simulink model "matlab_ros_com"  (R2017b)
settings: Solver=VariableStepAuto  StartTime=0.0  StopTime=inf  FixedStep=0.001  RelTol=1e-3  EnableMultiTasking=on
InitFcn:
  | sub_pose_time=0.1;
  | sub_vel_time=0.1;
  | pub_vel_time=0.1;
  | pub_pose_time=0.1;
undefined symbols (not defined in the file or in its folder): Pose, Twist
libraries: robotlib x28, simulink x5
settings Model: Creator=Administrator  LastModifiedBy=shitou
settings OptimizationCC: LifeSpan=inf
settings DebuggingCC: SFUnexpectedBacktrackingDiag=warning  SFNoUnconditionalDefaultTransitionDiag=warning  SFExecutionAtInitializationDiag=none
settings CodeAppCC: StateflowObjectComments=on
settings GRTTargetCC: TargetLangStandard=C89/C90 (ANSI)  GeneratePreprocessorConditionals=Disable all
settings ConfigComp: CovMetricSettings=dw  CovHtmlReporting=on  CovSaveCumulativeToWorkspaceVar=on  CovSaveSingleToWorkspaceVar=on  CovExternalEMLEnable=off

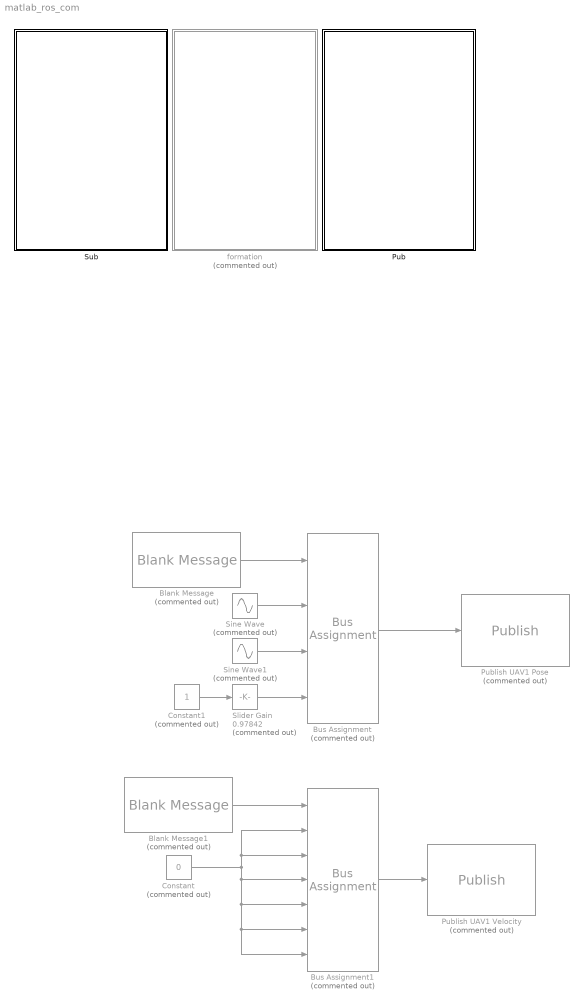
== system matlab_ros_com ==
  Blank Message : robotlib/Blank Message  Commented=on  SourceLibraryInfo=This block requires Robotics System Toolbox  messageType=geometry_msgs/PoseStamped  SampleTime=-1
      settings: SourceProductBaseCode=RO
  Blank Message1 : robotlib/Blank Message  Commented=on  SourceLibraryInfo=This block requires Robotics System Toolbox  messageType=geometry_msgs/TwistStamped  SampleTime=inf
      settings: SourceProductBaseCode=RO
  Bus Assignment : BusAssignment  Commented=on  AssignedSignals=Pose.Position.X,Pose.Position.Y,Pose.Position.Z
  Bus Assignment1 : BusAssignment  Commented=on  AssignedSignals=Twist.Linear.X,Twist.Linear.Y,Twist.Linear.Z,Twist.Angular.X,Twist.Angular.Y,Twist.Angular.Z
  Constant : Constant  Commented=on  Value=0
  Constant1 : Constant  Commented=on
  Pub : Subsystem
  Publish UAV1 Pose : robotlib/Publish  Commented=on  SourceLibraryInfo=This block requires Robotics System Toolbox  topicSource=Specify your own  topic=uav1_matlab/mavros/local_position/pose  messageType=geometry_msgs/PoseStamped  messageQueueLength=1
      settings: SourceProductBaseCode=RO
  Publish UAV1 Velocity : robotlib/Publish  Commented=on  SourceLibraryInfo=This block requires Robotics System Toolbox  topicSource=Specify your own  topic=uav1_matlab/mavros/local_position/velocity_local  messageType=geometry_msgs/TwistStamped  messageQueueLength=1
      settings: SourceProductBaseCode=RO
  Sine Wave : Sin  Commented=on  Frequency=0.05*pi
  Sine Wave1 : Sin  Commented=on  Frequency=0.05*pi  Phase=pi/2
  Slider Gain : simulink/Math Operations/Slider Gain  Commented=on  gain=0.97842  low=0  high=2
  Sub : Subsystem
  formation : Subsystem  Commented=on
  wires:
  Blank Message/1 -> Bus Assignment/1
  Bus Assignment/1 -> Publish UAV1 Pose/1
  Blank Message1/1 -> Bus Assignment1/1
  Bus Assignment1/1 -> Publish UAV1 Velocity/1
  Constant1/1 -> Slider Gain/1
  Slider Gain/1 -> Bus Assignment/4
  Sine Wave/1 -> Bus Assignment/2
  Sine Wave1/1 -> Bus Assignment/3
  Constant/1 -> Bus Assignment1/7, Bus Assignment1/6, Bus Assignment1/5, Bus Assignment1/4, Bus Assignment1/3, Bus Assignment1/2

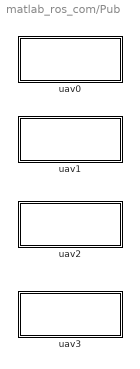
== system matlab_ros_com/Pub ==
  uav0 : Subsystem
  uav1 : Subsystem
  uav2 : Subsystem
  uav3 : Subsystem

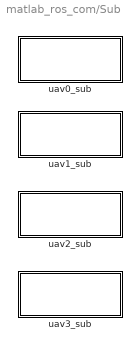
== system matlab_ros_com/Sub ==
  uav0_sub : Subsystem
  uav1_sub : Subsystem
  uav2_sub : Subsystem
  uav3_sub : Subsystem

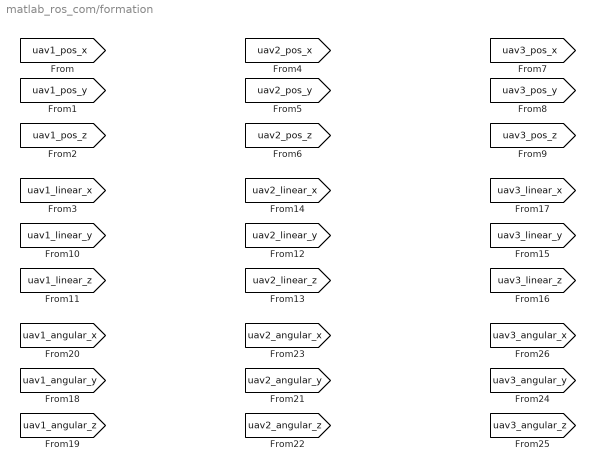
== system matlab_ros_com/formation ==

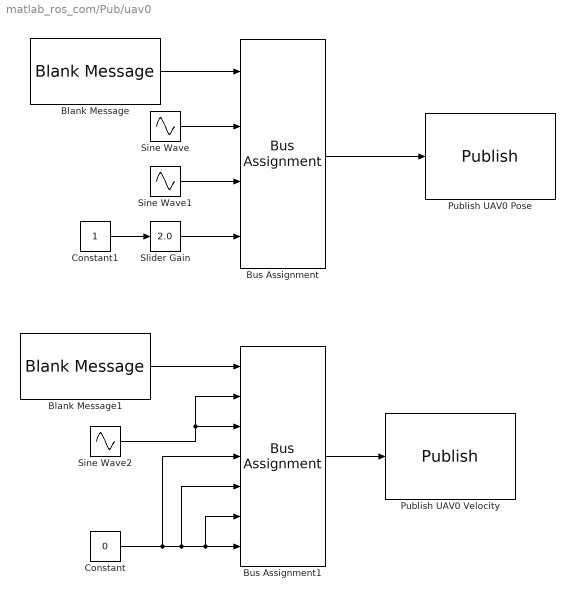
== system matlab_ros_com/Pub/uav0 ==
  Blank Message : robotlib/Blank Message  SourceLibraryInfo=This block requires Robotics System Toolbox  messageType=geometry_msgs/PoseStamped  SampleTime=pub_pose_time
      settings: SourceProductBaseCode=RO
  Blank Message1 : robotlib/Blank Message  SourceLibraryInfo=This block requires Robotics System Toolbox  messageType=geometry_msgs/TwistStamped  SampleTime=-1
      settings: SourceProductBaseCode=RO
  Bus Assignment : BusAssignment  AssignedSignals=Pose.Position.X,Pose.Position.Y,Pose.Position.Z
  Bus Assignment1 : BusAssignment  AssignedSignals=Twist.Linear.X,Twist.Linear.Y,Twist.Linear.Z,Twist.Angular.X,Twist.Angular.Y,Twist.Angular.Z
  Constant : Constant  Value=0  SampleTime=pub_vel_time
  Constant1 : Constant  SampleTime=pub_pose_time
  Publish UAV0 Pose : robotlib/Publish  SourceLibraryInfo=This block requires Robotics System Toolbox  topicSource=Specify your own  topic=uav0_matlab/mavros/local_position/pose  messageType=geometry_msgs/PoseStamped  messageQueueLength=1
      settings: SourceProductBaseCode=RO
  Publish UAV0 Velocity : robotlib/Publish  SourceLibraryInfo=This block requires Robotics System Toolbox  topicSource=Specify your own  topic=uav0_matlab/mavros/local_position/velocity_local  messageType=geometry_msgs/TwistStamped  messageQueueLength=1
      settings: SourceProductBaseCode=RO
  Sine Wave : Sin  Amplitude=10  Frequency=0.1*pi
  Sine Wave1 : Sin  Amplitude=10  Frequency=0.1*pi  Phase=pi/2
  Sine Wave2 : Sin  Frequency=0.1*pi  Phase=pi/2
  Slider Gain : simulink/Math Operations/Slider Gain  gain=2.0  low=0  high=2
  wires:
  Blank Message/1 -> Bus Assignment/1
  Bus Assignment/1 -> Publish UAV0 Pose/1
  Blank Message1/1 -> Bus Assignment1/1
  Bus Assignment1/1 -> Publish UAV0 Velocity/1
  Constant1/1 -> Slider Gain/1
  Slider Gain/1 -> Bus Assignment/4
  Sine Wave/1 -> Bus Assignment/2
  Sine Wave1/1 -> Bus Assignment/3
  Constant/1 -> Bus Assignment1/4, Bus Assignment1/5, Bus Assignment1/6, Bus Assignment1/7
  Sine Wave2/1 -> Bus Assignment1/3, Bus Assignment1/2

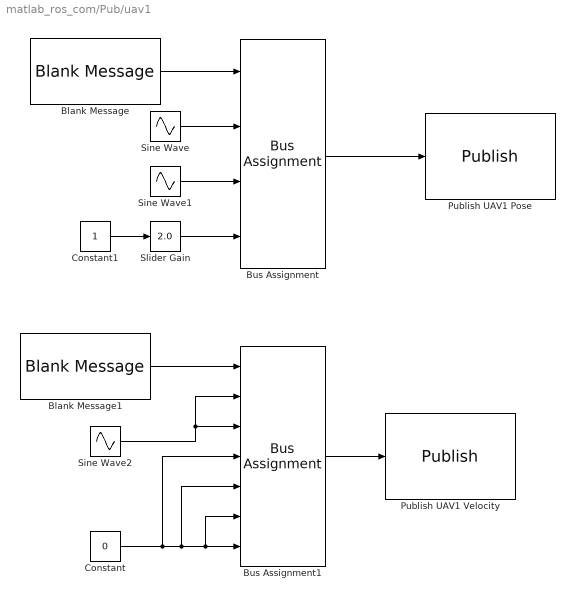
== system matlab_ros_com/Pub/uav1 ==
  Blank Message : robotlib/Blank Message  SourceLibraryInfo=This block requires Robotics System Toolbox  messageType=geometry_msgs/PoseStamped  SampleTime=pub_pose_time
      settings: SourceProductBaseCode=RO
  Blank Message1 : robotlib/Blank Message  SourceLibraryInfo=This block requires Robotics System Toolbox  messageType=geometry_msgs/TwistStamped  SampleTime=-1
      settings: SourceProductBaseCode=RO
  Bus Assignment : BusAssignment  AssignedSignals=Pose.Position.X,Pose.Position.Y,Pose.Position.Z
  Bus Assignment1 : BusAssignment  AssignedSignals=Twist.Linear.X,Twist.Linear.Y,Twist.Linear.Z,Twist.Angular.X,Twist.Angular.Y,Twist.Angular.Z
  Constant : Constant  Value=0  SampleTime=pub_vel_time
  Constant1 : Constant  SampleTime=pub_pose_time
  Publish UAV1 Pose : robotlib/Publish  SourceLibraryInfo=This block requires Robotics System Toolbox  topicSource=Specify your own  topic=uav1_matlab/mavros/local_position/pose  messageType=geometry_msgs/PoseStamped  messageQueueLength=1
      settings: SourceProductBaseCode=RO
  Publish UAV1 Velocity : robotlib/Publish  SourceLibraryInfo=This block requires Robotics System Toolbox  topicSource=Specify your own  topic=uav1_matlab/mavros/local_position/velocity_local  messageType=geometry_msgs/TwistStamped  messageQueueLength=1
      settings: SourceProductBaseCode=RO
  Sine Wave : Sin  Amplitude=10  Frequency=0.1*pi
  Sine Wave1 : Sin  Amplitude=10  Frequency=0.1*pi  Phase=pi/2
  Sine Wave2 : Sin  Frequency=0.1*pi  Phase=pi/2
  Slider Gain : simulink/Math Operations/Slider Gain  gain=2.0  low=0  high=2
  wires:
  Blank Message/1 -> Bus Assignment/1
  Bus Assignment/1 -> Publish UAV1 Pose/1
  Blank Message1/1 -> Bus Assignment1/1
  Bus Assignment1/1 -> Publish UAV1 Velocity/1
  Constant1/1 -> Slider Gain/1
  Slider Gain/1 -> Bus Assignment/4
  Sine Wave/1 -> Bus Assignment/2
  Sine Wave1/1 -> Bus Assignment/3
  Constant/1 -> Bus Assignment1/4, Bus Assignment1/5, Bus Assignment1/6, Bus Assignment1/7
  Sine Wave2/1 -> Bus Assignment1/3, Bus Assignment1/2

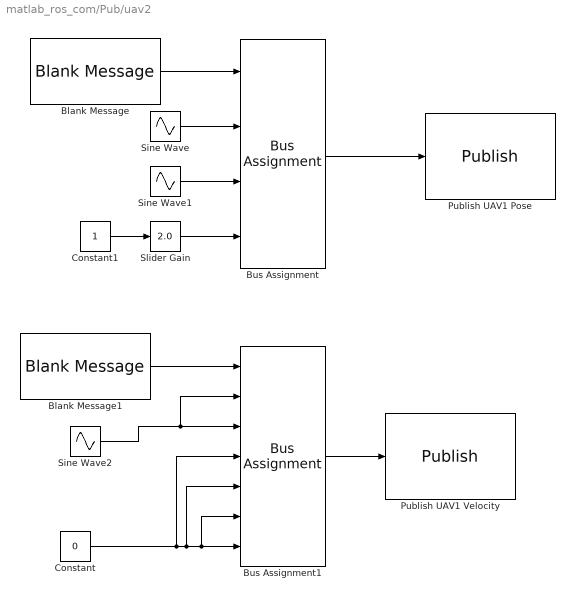
== system matlab_ros_com/Pub/uav2 ==
  Blank Message : robotlib/Blank Message  SourceLibraryInfo=This block requires Robotics System Toolbox  messageType=geometry_msgs/PoseStamped  SampleTime=pub_pose_time
      settings: SourceProductBaseCode=RO
  Blank Message1 : robotlib/Blank Message  SourceLibraryInfo=This block requires Robotics System Toolbox  messageType=geometry_msgs/TwistStamped  SampleTime=pub_vel_time
      settings: SourceProductBaseCode=RO
  Bus Assignment : BusAssignment  AssignedSignals=Pose.Position.X,Pose.Position.Y,Pose.Position.Z
  Bus Assignment1 : BusAssignment  AssignedSignals=Twist.Linear.X,Twist.Linear.Y,Twist.Linear.Z,Twist.Angular.X,Twist.Angular.Y,Twist.Angular.Z
  Constant : Constant  Value=0  SampleTime=pub_vel_time
  Constant1 : Constant  SampleTime=pub_pose_time
  Publish UAV1 Pose : robotlib/Publish  SourceLibraryInfo=This block requires Robotics System Toolbox  topicSource=Specify your own  topic=uav2_matlab/mavros/local_position/pose  messageType=geometry_msgs/PoseStamped  messageQueueLength=1
      settings: SourceProductBaseCode=RO
  Publish UAV1 Velocity : robotlib/Publish  SourceLibraryInfo=This block requires Robotics System Toolbox  topicSource=Specify your own  topic=uav2_matlab/mavros/local_position/velocity_local  messageType=geometry_msgs/TwistStamped  messageQueueLength=1
      settings: SourceProductBaseCode=RO
  Sine Wave : Sin  Amplitude=10  Frequency=0.1*pi
  Sine Wave1 : Sin  Amplitude=10  Frequency=0.1*pi  Phase=pi/2
  Sine Wave2 : Sin  Frequency=0.1*pi  Phase=pi/2
  Slider Gain : simulink/Math Operations/Slider Gain  gain=2.0  low=0  high=2
  wires:
  Blank Message/1 -> Bus Assignment/1
  Bus Assignment/1 -> Publish UAV1 Pose/1
  Blank Message1/1 -> Bus Assignment1/1
  Bus Assignment1/1 -> Publish UAV1 Velocity/1
  Constant1/1 -> Slider Gain/1
  Slider Gain/1 -> Bus Assignment/4
  Sine Wave/1 -> Bus Assignment/2
  Sine Wave1/1 -> Bus Assignment/3
  Constant/1 -> Bus Assignment1/4, Bus Assignment1/5, Bus Assignment1/6, Bus Assignment1/7
  Sine Wave2/1 -> Bus Assignment1/2, Bus Assignment1/3

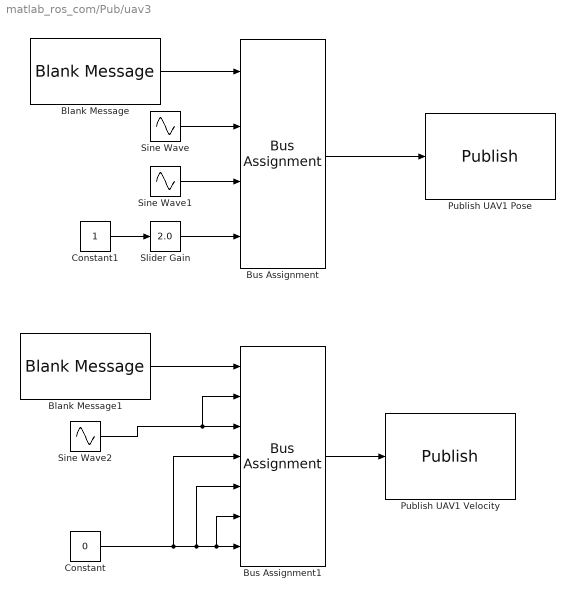
== system matlab_ros_com/Pub/uav3 ==
  Blank Message : robotlib/Blank Message  SourceLibraryInfo=This block requires Robotics System Toolbox  messageType=geometry_msgs/PoseStamped  SampleTime=pub_pose_time
      settings: SourceProductBaseCode=RO
  Blank Message1 : robotlib/Blank Message  SourceLibraryInfo=This block requires Robotics System Toolbox  messageType=geometry_msgs/TwistStamped  SampleTime=pub_vel_time
      settings: SourceProductBaseCode=RO
  Bus Assignment : BusAssignment  AssignedSignals=Pose.Position.X,Pose.Position.Y,Pose.Position.Z
  Bus Assignment1 : BusAssignment  AssignedSignals=Twist.Linear.X,Twist.Linear.Y,Twist.Linear.Z,Twist.Angular.X,Twist.Angular.Y,Twist.Angular.Z
  Constant : Constant  Value=0  SampleTime=pub_vel_time
  Constant1 : Constant  SampleTime=pub_pose_time
  Publish UAV1 Pose : robotlib/Publish  SourceLibraryInfo=This block requires Robotics System Toolbox  topicSource=Specify your own  topic=uav3_matlab/mavros/local_position/pose  messageType=geometry_msgs/PoseStamped  messageQueueLength=1
      settings: SourceProductBaseCode=RO
  Publish UAV1 Velocity : robotlib/Publish  SourceLibraryInfo=This block requires Robotics System Toolbox  topicSource=Specify your own  topic=uav3_matlab/mavros/local_position/velocity_local  messageType=geometry_msgs/TwistStamped  messageQueueLength=1
      settings: SourceProductBaseCode=RO
  Sine Wave : Sin  Amplitude=10  Frequency=0.1*pi
  Sine Wave1 : Sin  Amplitude=10  Frequency=0.1*pi  Phase=pi/2
  Sine Wave2 : Sin  Frequency=0.1*pi  Phase=pi/2
  Slider Gain : simulink/Math Operations/Slider Gain  gain=2.0  low=0  high=2
  wires:
  Blank Message/1 -> Bus Assignment/1
  Bus Assignment/1 -> Publish UAV1 Pose/1
  Blank Message1/1 -> Bus Assignment1/1
  Bus Assignment1/1 -> Publish UAV1 Velocity/1
  Constant1/1 -> Slider Gain/1
  Slider Gain/1 -> Bus Assignment/4
  Sine Wave/1 -> Bus Assignment/2
  Sine Wave1/1 -> Bus Assignment/3
  Constant/1 -> Bus Assignment1/4, Bus Assignment1/5, Bus Assignment1/6, Bus Assignment1/7
  Sine Wave2/1 -> Bus Assignment1/2, Bus Assignment1/3

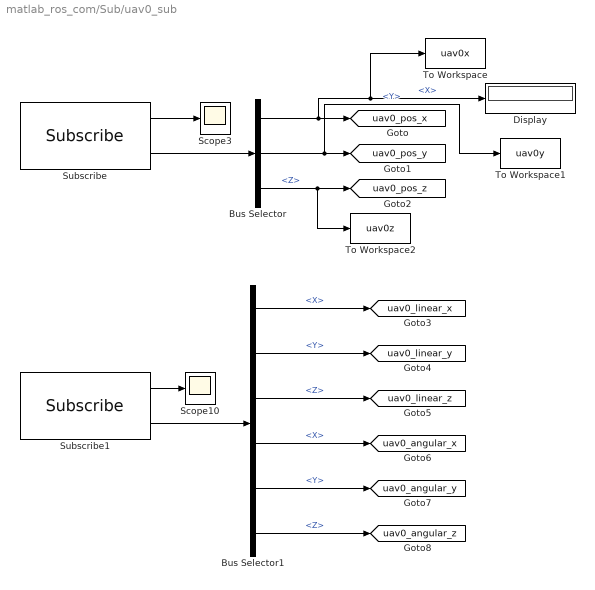
== system matlab_ros_com/Sub/uav0_sub ==
  Bus Selector : BusSelector  OutputSignals=Pose.Position.X,Pose.Position.Y,Pose.Position.Z
  Bus Selector1 : BusSelector  OutputSignals=Twist.Linear.X,Twist.Linear.Y,Twist.Linear.Z,Twist.Angular.X,Twist.Angular.Y,Twist.Angular.Z
  Display : Display
  Scope10 : Scope
  Scope3 : Scope
  Subscribe : robotlib/Subscribe  SourceLibraryInfo=This block requires Robotics System Toolbox  topicSource=Select from ROS network  topic=/uav0/mavros/local_position/pose  messageType=geometry_msgs/PoseStamped  sampleTime=sub_pose_time  messageQueueLength=1
      settings: SourceProductBaseCode=RO
  Subscribe1 : robotlib/Subscribe  SourceLibraryInfo=This block requires Robotics System Toolbox  topicSource=Select from ROS network  topic=/uav0/mavros/local_position/velocity_local  messageType=geometry_msgs/TwistStamped  sampleTime=sub_vel_time  messageQueueLength=1
      settings: SourceProductBaseCode=RO
  To Workspace : ToWorkspace  VariableName=uav0x  SaveFormat=Structure With Time  SampleTime=-1
  To Workspace1 : ToWorkspace  VariableName=uav0y  SaveFormat=Structure With Time  SampleTime=-1
  To Workspace2 : ToWorkspace  VariableName=uav0z  SaveFormat=Structure With Time  SampleTime=-1
  tag scope: uav0_angular_x=global, uav0_angular_y=global, uav0_angular_z=global, uav0_linear_x=global, uav0_linear_y=global, uav0_linear_z=global, uav0_pos_x=global, uav0_pos_y=global, uav0_pos_z=global
  wires:
  Subscribe/1 -> Scope3/1
  Subscribe/2 -> Bus Selector/1
  Bus Selector/1 -> To Workspace/1, Display/1, [uav0_pos_x]  "<X>"
  Bus Selector/2 -> To Workspace1/1, [uav0_pos_y]  "<Y>"
  Bus Selector/3 -> To Workspace2/1, [uav0_pos_z]  "<Z>"
  Subscribe1/2 -> Bus Selector1/1
  Subscribe1/1 -> Scope10/1
  Bus Selector1/1 -> [uav0_linear_x]  "<X>"
  Bus Selector1/2 -> [uav0_linear_y]  "<Y>"
  Bus Selector1/3 -> [uav0_linear_z]  "<Z>"
  Bus Selector1/4 -> [uav0_angular_x]  "<X>"
  Bus Selector1/5 -> [uav0_angular_y]  "<Y>"
  Bus Selector1/6 -> [uav0_angular_z]  "<Z>"

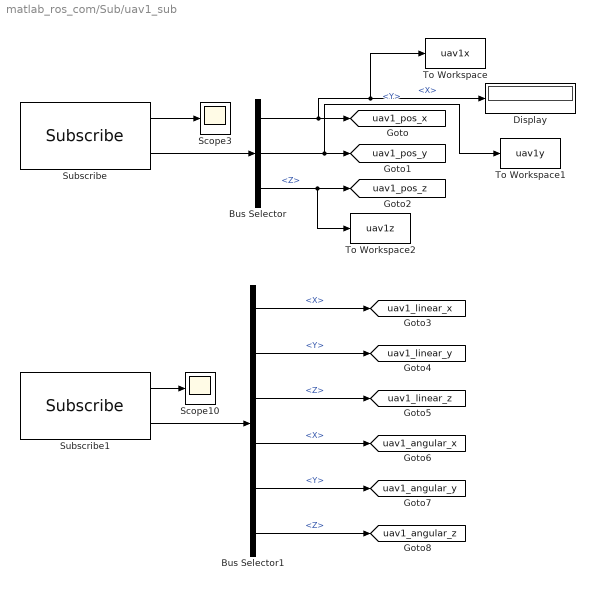
== system matlab_ros_com/Sub/uav1_sub ==
  Bus Selector : BusSelector  OutputSignals=Pose.Position.X,Pose.Position.Y,Pose.Position.Z
  Bus Selector1 : BusSelector  OutputSignals=Twist.Linear.X,Twist.Linear.Y,Twist.Linear.Z,Twist.Angular.X,Twist.Angular.Y,Twist.Angular.Z
  Display : Display
  Scope10 : Scope
  Scope3 : Scope
  Subscribe : robotlib/Subscribe  SourceLibraryInfo=This block requires Robotics System Toolbox  topicSource=Select from ROS network  topic=/uav1/mavros/local_position/pose  messageType=geometry_msgs/PoseStamped  sampleTime=sub_pose_time  messageQueueLength=1
      settings: SourceProductBaseCode=RO
  Subscribe1 : robotlib/Subscribe  SourceLibraryInfo=This block requires Robotics System Toolbox  topicSource=Select from ROS network  topic=/uav1/mavros/local_position/velocity_local  messageType=geometry_msgs/TwistStamped  sampleTime=sub_vel_time  messageQueueLength=1
      settings: SourceProductBaseCode=RO
  To Workspace : ToWorkspace  VariableName=uav1x  SaveFormat=Structure With Time  SampleTime=-1
  To Workspace1 : ToWorkspace  VariableName=uav1y  SaveFormat=Structure With Time  SampleTime=-1
  To Workspace2 : ToWorkspace  VariableName=uav1z  SaveFormat=Structure With Time  SampleTime=-1
  tag scope: uav1_angular_x=global, uav1_angular_y=global, uav1_angular_z=global, uav1_linear_x=global, uav1_linear_y=global, uav1_linear_z=global, uav1_pos_x=global, uav1_pos_y=global, uav1_pos_z=global
  wires:
  Subscribe/1 -> Scope3/1
  Subscribe/2 -> Bus Selector/1
  Bus Selector/1 -> To Workspace/1, Display/1, [uav1_pos_x]  "<X>"
  Bus Selector/2 -> To Workspace1/1, [uav1_pos_y]  "<Y>"
  Bus Selector/3 -> To Workspace2/1, [uav1_pos_z]  "<Z>"
  Subscribe1/2 -> Bus Selector1/1
  Subscribe1/1 -> Scope10/1
  Bus Selector1/1 -> [uav1_linear_x]  "<X>"
  Bus Selector1/2 -> [uav1_linear_y]  "<Y>"
  Bus Selector1/3 -> [uav1_linear_z]  "<Z>"
  Bus Selector1/4 -> [uav1_angular_x]  "<X>"
  Bus Selector1/5 -> [uav1_angular_y]  "<Y>"
  Bus Selector1/6 -> [uav1_angular_z]  "<Z>"

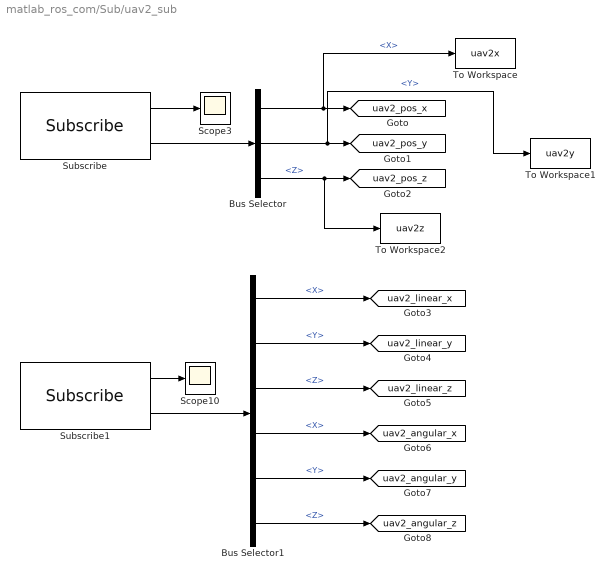
== system matlab_ros_com/Sub/uav2_sub ==
  Bus Selector : BusSelector  OutputSignals=Pose.Position.X,Pose.Position.Y,Pose.Position.Z
  Bus Selector1 : BusSelector  OutputSignals=Twist.Linear.X,Twist.Linear.Y,Twist.Linear.Z,Twist.Angular.X,Twist.Angular.Y,Twist.Angular.Z
  Scope10 : Scope
  Scope3 : Scope
  Subscribe : robotlib/Subscribe  SourceLibraryInfo=This block requires Robotics System Toolbox  topicSource=Select from ROS network  topic=/uav2/mavros/local_position/pose  messageType=geometry_msgs/PoseStamped  sampleTime=sub_pose_time  messageQueueLength=1
      settings: SourceProductBaseCode=RO
  Subscribe1 : robotlib/Subscribe  SourceLibraryInfo=This block requires Robotics System Toolbox  topicSource=Select from ROS network  topic=/uav2/mavros/local_position/velocity_local  messageType=geometry_msgs/TwistStamped  sampleTime=sub_vel_time  messageQueueLength=1
      settings: SourceProductBaseCode=RO
  To Workspace : ToWorkspace  VariableName=uav2x  SaveFormat=Structure With Time  SampleTime=-1
  To Workspace1 : ToWorkspace  VariableName=uav2y  SaveFormat=Structure With Time  SampleTime=-1
  To Workspace2 : ToWorkspace  VariableName=uav2z  SaveFormat=Structure With Time  SampleTime=-1
  tag scope: uav2_angular_x=global, uav2_angular_y=global, uav2_angular_z=global, uav2_linear_x=global, uav2_linear_y=global, uav2_linear_z=global, uav2_pos_x=global, uav2_pos_y=global, uav2_pos_z=global
  wires:
  Subscribe/1 -> Scope3/1
  Subscribe/2 -> Bus Selector/1
  Bus Selector/1 -> To Workspace/1, [uav2_pos_x]  "<X>"
  Bus Selector/2 -> To Workspace1/1, [uav2_pos_y]  "<Y>"
  Bus Selector/3 -> To Workspace2/1, [uav2_pos_z]  "<Z>"
  Subscribe1/2 -> Bus Selector1/1
  Subscribe1/1 -> Scope10/1
  Bus Selector1/1 -> [uav2_linear_x]  "<X>"
  Bus Selector1/2 -> [uav2_linear_y]  "<Y>"
  Bus Selector1/3 -> [uav2_linear_z]  "<Z>"
  Bus Selector1/4 -> [uav2_angular_x]  "<X>"
  Bus Selector1/5 -> [uav2_angular_y]  "<Y>"
  Bus Selector1/6 -> [uav2_angular_z]  "<Z>"

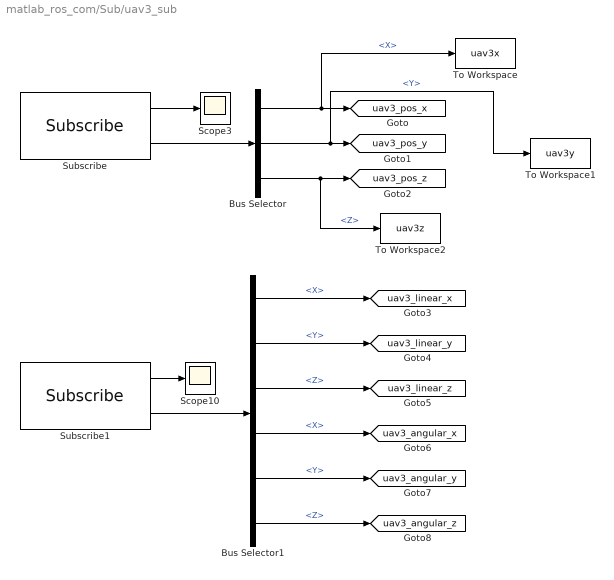
== system matlab_ros_com/Sub/uav3_sub ==
  Bus Selector : BusSelector  OutputSignals=Pose.Position.X,Pose.Position.Y,Pose.Position.Z
  Bus Selector1 : BusSelector  OutputSignals=Twist.Linear.X,Twist.Linear.Y,Twist.Linear.Z,Twist.Angular.X,Twist.Angular.Y,Twist.Angular.Z
  Scope10 : Scope
  Scope3 : Scope
  Subscribe : robotlib/Subscribe  SourceLibraryInfo=This block requires Robotics System Toolbox  topicSource=Select from ROS network  topic=/uav3/mavros/local_position/pose  messageType=geometry_msgs/PoseStamped  sampleTime=sub_pose_time  messageQueueLength=1
      settings: SourceProductBaseCode=RO
  Subscribe1 : robotlib/Subscribe  SourceLibraryInfo=This block requires Robotics System Toolbox  topicSource=Select from ROS network  topic=/uav3/mavros/local_position/velocity_local  messageType=geometry_msgs/TwistStamped  sampleTime=sub_vel_time  messageQueueLength=1
      settings: SourceProductBaseCode=RO
  To Workspace : ToWorkspace  VariableName=uav3x  SaveFormat=Structure With Time  SampleTime=-1
  To Workspace1 : ToWorkspace  VariableName=uav3y  SaveFormat=Structure With Time  SampleTime=-1
  To Workspace2 : ToWorkspace  VariableName=uav3z  SaveFormat=Structure With Time  SampleTime=-1
  tag scope: uav3_angular_x=global, uav3_angular_y=global, uav3_angular_z=global, uav3_linear_x=global, uav3_linear_y=global, uav3_linear_z=global, uav3_pos_x=global, uav3_pos_y=global, uav3_pos_z=global
  wires:
  Subscribe/1 -> Scope3/1
  Subscribe/2 -> Bus Selector/1
  Bus Selector/1 -> To Workspace/1, [uav3_pos_x]  "<X>"
  Bus Selector/2 -> To Workspace1/1, [uav3_pos_y]  "<Y>"
  Bus Selector/3 -> To Workspace2/1, [uav3_pos_z]  "<Z>"
  Subscribe1/2 -> Bus Selector1/1
  Subscribe1/1 -> Scope10/1
  Bus Selector1/1 -> [uav3_linear_x]  "<X>"
  Bus Selector1/2 -> [uav3_linear_y]  "<Y>"
  Bus Selector1/3 -> [uav3_linear_z]  "<Z>"
  Bus Selector1/4 -> [uav3_angular_x]  "<X>"
  Bus Selector1/5 -> [uav3_angular_y]  "<Y>"
  Bus Selector1/6 -> [uav3_angular_z]  "<Z>"
